simulink model "FRC_0"  (R2018b)
settings: Solver=VariableStepAuto  StartTime=0.0  StopTime=500000.0  RelTol=1e-3
libraries: simulink x1
(part 1 of 2)
settings Model: Creator=user  LastModifiedBy=user

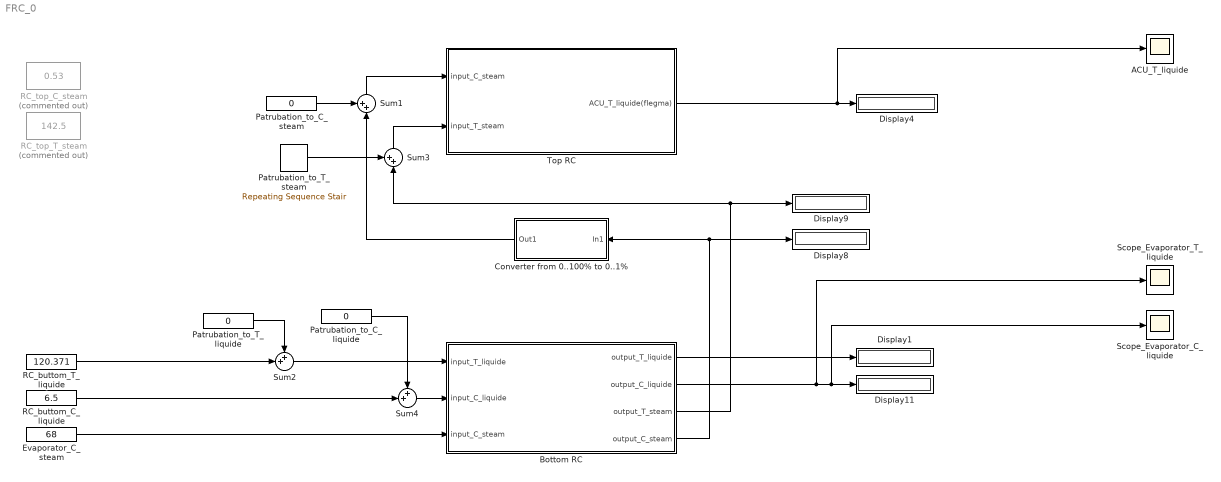
== system FRC_0 ==
  ACU_T_liquide : Scope
  Bottom RC : Subsystem
  Converter from 0..100% to 0..1% : Subsystem
  Display{1,4,8..9,11} (5 alike) : Display
  Evaporator_C_steam : Constant  Value=68
  Patrubation_to_C_liquide : Constant  Value=0
  Patrubation_to_C_steam : Constant  Value=0
  Patrubation_to_T_liquide : Constant  Value=0
  Patrubation_to_T_steam : simulink/Sources/Repeating Sequence Stair  OutValues=[0 0 0 0 0 0 0 0 0 0 2 2 2 2 2 2 2 2].'  tsamp=-1  OutMin=[]  OutMax=[]  OutDataTypeStr=double  OutputDataTypeScalingMode=double  OutDataType=fixdt(0,8)  ConRadixGroup=Best Precision: Vector-wise  OutScaling=2^-12
  RC_buttom_C_liquide : Constant  Value=6.5
  RC_buttom_T_liquide : Constant  Value=120.371
  RC_top_C_steam : Constant  Commented=on  Value=0.53
  RC_top_T_steam : Constant  Commented=on  Value=142.5
  Scope_Evaporator_C_liquide : Scope
  Scope_Evaporator_T_liquide : Scope
  Sum{1..4} (4 alike) : Sum  Inputs=++|
  Top RC : Subsystem
  wires:
  Top RC/1(ACU_T_liquide(flegma)) -> ACU_T_liquide/1, Display4/1
  Bottom RC/2(output_C_liquide) -> Scope_Evaporator_T_liquide/1, Scope_Evaporator_C_liquide/1, Display11/1
  RC_buttom_C_liquide/1 -> Sum4/2
  Evaporator_C_steam/1 -> Bottom RC/3(input_C_steam)
  RC_buttom_T_liquide/1 -> Sum2/2
  Bottom RC/4(output_C_steam) -> Converter from 0..100% to 0..1%/1(In1), Display8/1
  Bottom RC/3(output_T_steam) -> Sum3/2, Display9/1
  Bottom RC/1(output_T_liquide) -> Display1/1
  Converter from 0..100% to 0..1%/1(Out1) -> Sum1/2
  Sum3/1 -> Top RC/2(input_T_steam)
  Patrubation_to_C_steam/1 -> Sum1/1
  Sum1/1 -> Top RC/1(input_C_steam)
  Sum2/1 -> Bottom RC/1(input_T_liquide)
  Patrubation_to_T_liquide/1 -> Sum2/1
  Patrubation_to_C_liquide/1 -> Sum4/1
  Sum4/1 -> Bottom RC/2(input_C_liquide)
  Patrubation_to_T_steam/1 -> Sum3/1

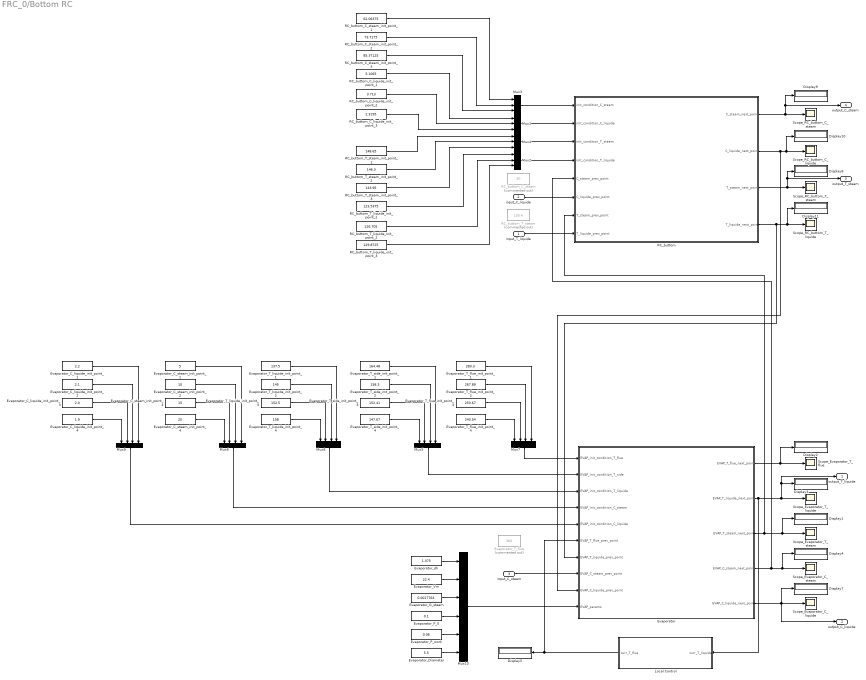
== system FRC_0/Bottom RC ==
  input_T_liquide : Inport
  input_C_liquide : Inport  Port=2
  input_C_steam : Inport  Port=3
  Display{1..5,7..11} (10 alike) : Display
  Evaporator : Subsystem
  Evaporator_C_liquide_init_point_1 : Constant  Value=2.2
  Evaporator_C_liquide_init_point_2 : Constant  Value=2.1
  Evaporator_C_liquide_init_point_3 : Constant  Value=2.0
  Evaporator_C_liquide_init_point_4 : Constant  Value=1.9
  Evaporator_C_steam_init_point_1 : Constant  Value=5
  Evaporator_C_steam_init_point_2 : Constant  Value=10
  Evaporator_C_steam_init_point_3 : Constant  Value=15
  Evaporator_C_steam_init_point_4 : Constant  Value=20
  Evaporator_Diameter : Constant  Value=5.5
  Evaporator_G_steam : Constant  Value=0.0017763
  Evaporator_P_0 : Constant  Value=0.1
  Evaporator_P_work : Constant  Value=0.06
  Evaporator_T_flue : Constant  Commented=on  Value=360
  Evaporator_T_flue_init_point_1 : Constant  Value=283.3
  Evaporator_T_flue_init_point_2 : Constant  Value=267.89
  Evaporator_T_flue_init_point_3 : Constant  Value=253.67
  Evaporator_T_flue_init_point_4 : Constant  Value=240.54
  Evaporator_T_liquide_init_point_1 : Constant  Value=137.5
  Evaporator_T_liquide_init_point_2 : Constant  Value=145
  Evaporator_T_liquide_init_point_3 : Constant  Value=152.5
  Evaporator_T_liquide_init_point_4 : Constant  Value=158
  Evaporator_T_side_init_point_1 : Constant  Value=164.48
  Evaporator_T_side_init_point_2 : Constant  Value=158.3
  Evaporator_T_side_init_point_3 : Constant  Value=152.41
  Evaporator_T_side_init_point_4 : Constant  Value=147.07
  Evaporator_Vm : Constant  Value=22.4
  Evaporator_dh : Constant  Value=1.375
  Local Control : Subsystem
  Mux{1..4} (4 alike) : Mux  Inputs=3
  Mux10 : Mux  Inputs=6
  Mux{5..9} (5 alike) : Mux
  RC_buttom : Subsystem
  RC_buttom_C_liquide_init_point_1 : Constant  Value=5.1065
  RC_buttom_C_liquide_init_point_2 : Constant  Value=3.713
  RC_buttom_C_liquide_init_point_3 : Constant  Value=2.3195
  RC_buttom_C_steam : Constant  Commented=on  Value=50
  RC_buttom_C_steam_init_point_1 : Constant  Value=62.06375
  RC_buttom_C_steam_init_point_2 : Constant  Value=73.7175
  RC_buttom_C_steam_init_point_3 : Constant  Value=85.37125
  RC_buttom_T_liquide_init_point_1 : Constant  Value=123.5375
  RC_buttom_T_liquide_init_point_2 : Constant  Value=126.705
  RC_buttom_T_liquide_init_point_3 : Constant  Value=129.8725
  RC_buttom_T_steam : Constant  Commented=on  Value=150.4
  RC_buttom_T_steam_init_point_1 : Constant  Value=148.65
  RC_buttom_T_steam_init_point_2 : Constant  Value=146.3
  RC_buttom_T_steam_init_point_3 : Constant  Value=143.95
  Scope_Evaporator_C_liquide : Scope
  Scope_Evaporator_C_steam : Scope
  Scope_Evaporator_T_flue : Scope
  Scope_Evaporator_T_liquide : Scope
  Scope_Evaporator_T_steam : Scope
  Scope_RC_buttom_C_liquide : Scope
  Scope_RC_buttom_C_steam : Scope
  Scope_RC_buttom_T_liquide : Scope
  Scope_RC_buttom_T_steam : Scope
  output_T_liquide : Outport
  output_C_liquide : Outport  Port=2
  output_T_steam : Outport  Port=3
  output_C_steam : Outport  Port=4
  wires:
  Evaporator_T_side_init_point_3/1 -> Mux5/2
  Evaporator_C_steam_init_point_2/1 -> Mux6/3
  Evaporator_C_liquide_init_point_1/1 -> Mux9/4
  RC_buttom_T_steam_init_point_1/1 -> Mux4/1
  Evaporator_C_steam_init_point_4/1 -> Mux6/1
  RC_buttom_C_steam_init_point_1/1 -> Mux3/1
  Mux1/1 -> RC_buttom/2(init_condition_C_liquide)
  Evaporator_T_liquide_init_point_4/1 -> Mux8/1
  Evaporator_C_steam_init_point_3/1 -> Mux6/2
  Evaporator/2(EVAP_T_liquide_next_point) -> Local Control/1(curr_T_liquide), output_T_liquide/1, Display3/1, Scope_Evaporator_T_liquide/1
  RC_buttom/4(T_liquide_next_point) -> Evaporator/7(EVAP_T_liquide_prev_point), Display11/1, Scope_RC_buttom_T_liquide/1
  Evaporator_C_liquide_init_point_2/1 -> Mux9/3
  Evaporator_G_steam/1 -> Mux10/3
  Local Control/1(curr_T_flue) -> Evaporator/6(EVAP_T_flue_prev_point), Display5/1
  Mux8/1 -> Evaporator/3(EVAP_init_condition_T_liquide)
  Evaporator_P_0/1 -> Mux10/4
  Mux6/1 -> Evaporator/4(EVAP_init_condition_C_steam)
  Evaporator_T_flue_init_point_2/1 -> Mux7/3
  RC_buttom_C_liquide_init_point_2/1 -> Mux1/2
  Evaporator_P_work/1 -> Mux10/5
  RC_buttom_T_steam_init_point_3/1 -> Mux4/3
  Evaporator_C_liquide_init_point_3/1 -> Mux9/2
  Evaporator_C_liquide_init_point_4/1 -> Mux9/1
  input_T_liquide/1 -> RC_buttom/8(T_liquide_prev_point)
  Mux4/1 -> RC_buttom/3(init_condition_T_steam)
  Evaporator/1(EVAP_T_flue_next_point) -> Display2/1, Scope_Evaporator_T_flue/1
  Evaporator_T_flue_init_point_4/1 -> Mux7/1
  RC_buttom/3(T_steam_next_point) -> output_T_steam/1, Display8/1, Scope_RC_buttom_T_steam/1
  Evaporator/3(EVAP_T_steam_next_point) -> Display1/1, Scope_Evaporator_T_steam/1, RC_buttom/7(T_steam_prev_point)
  RC_buttom_C_liquide_init_point_1/1 -> Mux1/1
  Evaporator_T_flue_init_point_1/1 -> Mux7/4
  RC_buttom/2(C_liquide_next_point) -> Display10/1, Scope_RC_buttom_C_liquide/1, Evaporator/9(EVAP_C_liquide_prev_point)
  Evaporator/5(EVAP_C_liquide_next_point) -> output_C_liquide/1, Display7/1, Scope_Evaporator_C_liquide/1
  Mux3/1 -> RC_buttom/1(init_condition_C_steam)
  Evaporator_T_side_init_point_1/1 -> Mux5/4
  RC_buttom_T_steam_init_point_2/1 -> Mux4/2
  RC_buttom_C_steam_init_point_2/1 -> Mux3/2
  Evaporator_T_side_init_point_2/1 -> Mux5/3
  RC_buttom_T_liquide_init_point_1/1 -> Mux2/1
  Evaporator_T_side_init_point_4/1 -> Mux5/1
  Evaporator_T_flue_init_point_3/1 -> Mux7/2
  RC_buttom_C_liquide_init_point_3/1 -> Mux1/3
  Evaporator_T_liquide_init_point_1/1 -> Mux8/4
  RC_buttom_T_liquide_init_point_3/1 -> Mux2/3
  RC_buttom/1(C_steam_next_point) -> Display9/1, output_C_steam/1, Scope_RC_buttom_C_steam/1
  Evaporator_T_liquide_init_point_2/1 -> Mux8/3
  Evaporator_Vm/1 -> Mux10/2
  Mux7/1 -> Evaporator/1(EVAP_init_condition_T_flue)
  RC_buttom_T_liquide_init_point_2/1 -> Mux2/2
  Mux5/1 -> Evaporator/2(EVAP_init_condition_T_side)
  input_C_steam/1 -> Evaporator/8(EVAP_C_steam_prev_point)
  Mux2/1 -> RC_buttom/4(init_condition_T_liquide)
  Evaporator/4(EVAP_C_steam_next_point) -> RC_buttom/5(C_steam_prev_point), Display4/1, Scope_Evaporator_C_steam/1
  Mux10/1 -> Evaporator/10(EVAP_params)
  Evaporator_C_steam_init_point_1/1 -> Mux6/4
  Evaporator_T_liquide_init_point_3/1 -> Mux8/2
  Mux9/1 -> Evaporator/5(EVAP_init_condition_C_liquide)
  RC_buttom_C_steam_init_point_3/1 -> Mux3/3
  Evaporator_dh/1 -> Mux10/1
  Evaporator_Diameter/1 -> Mux10/6
  input_C_liquide/1 -> RC_buttom/6(C_liquide_prev_point)

== system FRC_0/Converter from 0..100% to 0..1% ==
  In1 : Inport
  Converter from 0..100% to 0..1% : Gain  Gain=0.01
  Out1 : Outport
  wires:
  In1/1 -> Converter from 0..100% to 0..1%/1
  Converter from 0..100% to 0..1%/1 -> Out1/1

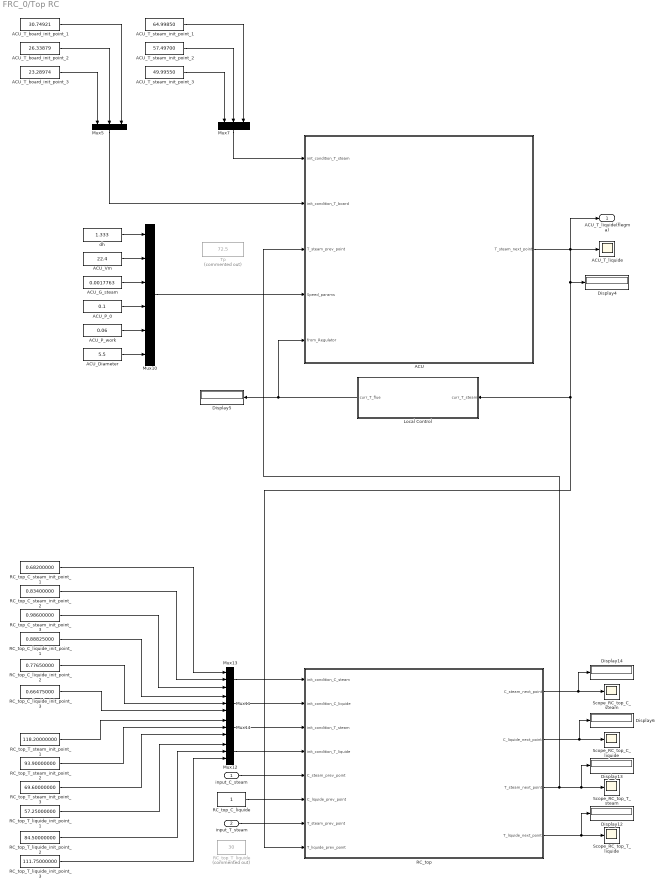
== system FRC_0/Top RC ==
  input_C_steam : Inport
  input_T_steam : Inport  Port=2
  ACU : Subsystem
  ACU_Diameter : Constant  Value=5.5
  ACU_G_steam : Constant  Value=0.0017763
  ACU_P_0 : Constant  Value=0.1
  ACU_P_work : Constant  Value=0.06
  ACU_T_board_init_point_1 : Constant  Value=30.74921
  ACU_T_board_init_point_2 : Constant  Value=26.33879
  ACU_T_board_init_point_3 : Constant  Value=23.28974
  ACU_T_liquide : Scope
  ACU_T_steam_init_point_1 : Constant  Value=64.99850
  ACU_T_steam_init_point_2 : Constant  Value=57.49700
  ACU_T_steam_init_point_3 : Constant  Value=49.99550
  ACU_Vm : Constant  Value=22.4
  Display{4..6,12..14} (6 alike) : Display
  Local Control : Subsystem
  Mux10 : Mux  Inputs=6
  Mux{5,7,11..14} (6 alike) : Mux  Inputs=3
  RC_top : Subsystem
  RC_top_C_liquide : Constant
  RC_top_C_liquide_init_point_1 : Constant  Value=0.88825000
  RC_top_C_liquide_init_point_2 : Constant  Value=0.77650000
  RC_top_C_liquide_init_point_3 : Constant  Value=0.66475000
  RC_top_C_steam_init_point_1 : Constant  Value=0.68200000
  RC_top_C_steam_init_point_2 : Constant  Value=0.83400000
  RC_top_C_steam_init_point_3 : Constant  Value=0.98600000
  RC_top_T_liquide : Constant  Commented=on  Value=30
  RC_top_T_liquide_init_point_1 : Constant  Value=57.25000000
  RC_top_T_liquide_init_point_2 : Constant  Value=84.50000000
  RC_top_T_liquide_init_point_3 : Constant  Value=111.75000000
  RC_top_T_steam_init_point_1 : Constant  Value=118.20000000
  RC_top_T_steam_init_point_2 : Constant  Value=93.90000000
  RC_top_T_steam_init_point_3 : Constant  Value=69.60000000
  Scope_RC_top_C_liquide : Scope
  Scope_RC_top_C_steam : Scope
  Scope_RC_top_T_liquide : Scope
  Scope_RC_top_T_steam : Scope
  Tp : Constant  Commented=on  Value=72.5
  dh : Constant  Value=1.333
  ACU_T_liquide(flegma) : Outport
  wires:
  RC_top_C_steam_init_point_3/1 -> Mux13/3
  RC_top_T_steam_init_point_3/1 -> Mux14/3
  RC_top_T_liquide_init_point_2/1 -> Mux12/2
  RC_top_C_steam_init_point_2/1 -> Mux13/2
  RC_top_C_liquide_init_point_2/1 -> Mux11/2
  RC_top_T_liquide_init_point_1/1 -> Mux12/1
  RC_top/1(C_steam_next_point) -> Display14/1, Scope_RC_top_C_steam/1
  RC_top_C_liquide_init_point_1/1 -> Mux11/1
  Mux14/1 -> RC_top/3(init_condition_T_steam)
  RC_top_C_liquide/1 -> RC_top/6(C_liquide_prev_point)
  RC_top/2(C_liquide_next_point) -> Display6/1, Scope_RC_top_C_liquide/1
  Mux12/1 -> RC_top/4(init_condition_T_liquide)
  RC_top_T_steam_init_point_2/1 -> Mux14/2
  Mux13/1 -> RC_top/1(init_condition_C_steam)
  RC_top_T_liquide_init_point_3/1 -> Mux12/3
  RC_top_T_steam_init_point_1/1 -> Mux14/1
  RC_top_C_liquide_init_point_3/1 -> Mux11/3
  Mux11/1 -> RC_top/2(init_condition_C_liquide)
  RC_top_C_steam_init_point_1/1 -> Mux13/1
  RC_top/4(T_liquide_next_point) -> Display12/1, Scope_RC_top_T_liquide/1
  Mux5/1 -> ACU/2(init_condition_T_board)
  ACU_Vm/1 -> Mux10/2
  Mux7/1 -> ACU/1(init_condition_T_steam)
  ACU_G_steam/1 -> Mux10/3
  ACU_P_work/1 -> Mux10/5
  Local Control/1(curr_T_flue) -> ACU/5(from_Regulator), Display5/1
  ACU_P_0/1 -> Mux10/4
  Mux10/1 -> ACU/4(Speed_params)
  dh/1 -> Mux10/1
  ACU_Diameter/1 -> Mux10/6
  input_C_steam/1 -> RC_top/5(C_steam_prev_point)
  input_T_steam/1 -> RC_top/7(T_steam_prev_point)
  ACU_T_steam_init_point_1/1 -> Mux7/3
  ACU_T_steam_init_point_2/1 -> Mux7/2
  ACU_T_steam_init_point_3/1 -> Mux7/1
  ACU_T_board_init_point_1/1 -> Mux5/3
  ACU_T_board_init_point_2/1 -> Mux5/2
  ACU_T_board_init_point_3/1 -> Mux5/1
  RC_top/3(T_steam_next_point) -> ACU/3(T_steam_prev_point), Display13/1, Scope_RC_top_T_steam/1
  ACU/1(T_steam_next_point) -> ACU_T_liquide(flegma)/1, RC_top/8(T_liquide_prev_point), Local Control/1(curr_T_steam), Display4/1, ACU_T_liquide/1

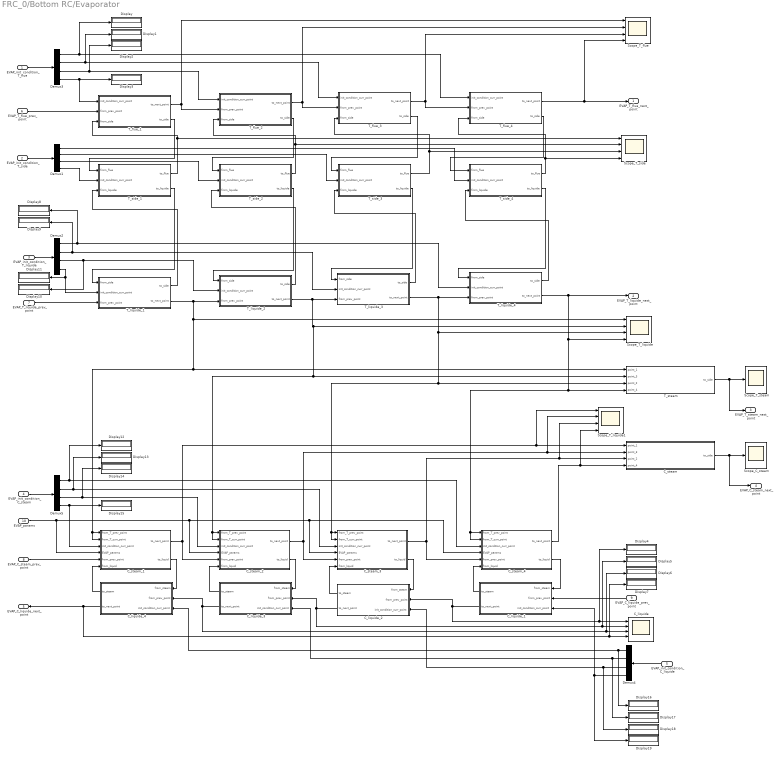
== system FRC_0/Bottom RC/Evaporator ==
  EVAP_init_condition_T_flue : Inport
  EVAP_init_condition_T_side : Inport  Port=2
  EVAP_init_condition_T_liquide : Inport  Port=3
  EVAP_init_condition_C_steam : Inport  Port=4
  EVAP_init_condition_C_liquide : Inport  Port=5
  EVAP_T_flue_prev_point : Inport  Port=6
  EVAP_T_liquide_prev_point : Inport  Port=7
  EVAP_C_steam_prev_point : Inport  Port=8
  EVAP_C_liquide_prev_point : Inport  Port=9
  EVAP_params : Inport  Port=10
  C_liquide : Scope  NumInputPorts=4
  C_liquide_1 : Subsystem
  C_liquide_2 : Subsystem
  C_liquide_3 : Subsystem
  C_liquide_4 : Subsystem
  C_steam : Subsystem
  C_steam_1 : Subsystem
  C_steam_2 : Subsystem
  C_steam_3 : Subsystem
  C_steam_4 : Subsystem
  Demux{1..5} (5 alike) : Demux
  Display{,1..19} (20 alike) : Display
  Scope_C_steam : Scope
  Scope_T_flue : Scope  NumInputPorts=4
  Scope_T_liquide : Scope  NumInputPorts=4
  Scope_T_liquide1 : Scope  NumInputPorts=4
  Scope_T_side : Scope  NumInputPorts=4
  Scope_T_steam : Scope
  T_flue_1 : Subsystem
  T_flue_2 : Subsystem
  T_flue_3 : Subsystem
  T_flue_4 : Subsystem
  T_liquide_1 : Subsystem
  T_liquide_2 : Subsystem
  T_liquide_3 : Subsystem
  T_liquide_4 : Subsystem
  T_side_1 : Subsystem
  T_side_2 : Subsystem
  T_side_3 : Subsystem
  T_side_4 : Subsystem
  T_steam : Subsystem
  EVAP_T_flue_next_point : Outport
  EVAP_T_liquide_next_point : Outport  Port=2
  EVAP_T_steam_next_point : Outport  Port=3
  EVAP_C_steam_next_point : Outport  Port=4
  EVAP_C_liquide_next_point : Outport  Port=5
  wires:
  T_liquide_3/2(to_next_point) -> T_liquide_4/3(from_prev_point), C_steam_3/1(from_T_prev_point), C_steam_3/2(from_T_curr_point), T_steam/3(point_2), Scope_T_liquide/3
  EVAP_init_condition_T_liquide/1 -> Demux2/1
  Demux2/1 -> T_liquide_4/2(init_condition_curr_point), Display8/1
  EVAP_init_condition_T_side/1 -> Demux1/1
  T_liquide_4/2(to_next_point) -> Scope_T_liquide/4, C_steam_4/2(from_T_curr_point), C_steam_4/1(from_T_prev_point), T_steam/4(point_4), EVAP_T_liquide_next_point/1
  Demux2/2 -> T_liquide_3/2(init_condition_curr_point), Display9/1
  Demux2/4 -> T_liquide_1/2(init_condition_curr_point), Display11/1
  EVAP_init_condition_T_flue/1 -> Demux3/1
  T_flue_1/1(to_next_point) -> T_flue_2/2(from_prev_point), Scope_T_flue/1
  T_flue_2/1(to_next_point) -> T_flue_3/2(from_prev_point), Scope_T_flue/2
  T_flue_3/1(to_next_point) -> T_flue_4/2(from_prev_point), Scope_T_flue/3
  Demux3/1 -> T_flue_4/1(init_condition_curr_point), Display/1
  Demux3/2 -> T_flue_3/1(init_condition_curr_point), Display1/1
  Demux3/3 -> T_flue_2/1(init_condition_curr_point), Display2/1
  Demux3/4 -> T_flue_1/1(init_condition_curr_point), Display3/1
  T_flue_4/1(to_next_point) -> EVAP_T_flue_next_point/1, Scope_T_flue/4
  EVAP_T_flue_prev_point/1 -> T_flue_1/2(from_prev_point)
  T_steam/1(to_side) -> EVAP_T_steam_next_point/1, Scope_T_steam/1
  Demux5/2 -> C_steam_3/3(init_condition_curr_point), Display13/1
  C_liquide_2/2(to_next_point) -> C_liquide_3/2(from_prev_point), Display5/1, C_liquide/2
  C_steam_2/1(to_next_point) -> C_steam_3/5(from_prev_point), Scope_T_liquide1/2, C_steam/2(point_3)
  EVAP_init_condition_C_liquide/1 -> Demux4/1
  Demux5/3 -> C_steam_2/3(init_condition_curr_point), Display14/1
  C_steam_1/2(to_liquid) -> C_liquide_4/1(from_steam)
  Demux5/1 -> C_steam_4/3(init_condition_curr_point), Display12/1
  EVAP_init_condition_C_steam/1 -> Demux5/1
  EVAP_C_steam_prev_point/1 -> C_steam_1/5(from_prev_point)
  C_liquide_4/2(to_next_point) -> EVAP_C_liquide_next_point/1, Display7/1, C_liquide/4
  C_liquide_2/1(to_steam) -> C_steam_3/6(from_liquid)
  C_liquide_3/2(to_next_point) -> C_liquide_4/2(from_prev_point), Display6/1, C_liquide/3
  C_liquide_4/1(to_steam) -> C_steam_1/6(from_liquid)
  C_steam_3/1(to_next_point) -> C_steam_4/5(from_prev_point), Scope_T_liquide1/3, C_steam/3(point_2)
  EVAP_C_liquide_prev_point/1 -> C_liquide_1/2(from_prev_point)
  C_steam_4/2(to_liquid) -> C_liquide_1/1(from_steam)
  C_liquide_1/1(to_steam) -> C_steam_4/6(from_liquid)
  Demux5/4 -> C_steam_1/3(init_condition_curr_point), Display15/1
  C_liquide_1/2(to_next_point) -> C_liquide_2/2(from_prev_point), Display4/1, C_liquide/1
  Demux4/1 -> C_liquide_4/3(init_condition_curr_point), Display16/1
  Demux4/2 -> C_liquide_3/3(init_condition_curr_point), Display17/1
  Demux4/3 -> C_liquide_2/3(init_condition_curr_point), Display18/1
  Demux4/4 -> C_liquide_1/3(init_condition_curr_point), Display19/1
  C_steam/1(to_side) -> EVAP_C_steam_next_point/1, Scope_C_steam/1
  C_steam_1/1(to_next_point) -> C_steam_2/5(from_prev_point), Scope_T_liquide1/1, C_steam/1(point_1)
  C_steam_4/1(to_next_point) -> Scope_T_liquide1/4, C_steam/4(point_4)
  EVAP_params/1 -> C_steam_1/4(EVAP_params), C_steam_2/4(EVAP_params), C_steam_4/4(EVAP_params), C_steam_3/4(EVAP_params)
  C_liquide_3/1(to_steam) -> C_steam_2/6(from_liquid)
  C_steam_2/2(to_liquid) -> C_liquide_3/1(from_steam)
  EVAP_T_liquide_prev_point/1 -> T_liquide_1/3(from_prev_point)
  C_steam_3/2(to_liquid) -> C_liquide_2/1(from_steam)
  T_liquide_1/2(to_next_point) -> T_liquide_2/3(from_prev_point), Scope_T_liquide/1, T_steam/1(point_1), C_steam_1/1(from_T_prev_point), C_steam_1/2(from_T_curr_point)
  Demux2/3 -> T_liquide_2/2(init_condition_curr_point), Display10/1
  T_side_1/1(to_flue) -> Scope_T_side/1, T_flue_1/3(from_side)
  T_flue_1/2(to_side) -> T_side_1/1(from_flue)
  T_side_1/2(to_liquide) -> T_liquide_1/1(from_side)
  T_liquide_1/1(to_side) -> T_side_1/3(from_liquide)
  Demux1/4 -> T_side_1/2(init_condition_curr_point)
  T_side_2/1(to_flue) -> T_flue_2/3(from_side), Scope_T_side/2
  T_flue_2/2(to_side) -> T_side_2/1(from_flue)
  T_side_3/1(to_flue) -> T_flue_3/3(from_side), Scope_T_side/3
  T_flue_3/2(to_side) -> T_side_3/1(from_flue)
  T_side_4/1(to_flue) -> T_flue_4/3(from_side), Scope_T_side/4
  T_flue_4/2(to_side) -> T_side_4/1(from_flue)
  T_liquide_2/1(to_side) -> T_side_2/3(from_liquide)
  T_side_2/2(to_liquide) -> T_liquide_2/1(from_side)
  T_side_3/2(to_liquide) -> T_liquide_3/1(from_side)
  T_liquide_3/1(to_side) -> T_side_3/3(from_liquide)
  T_side_4/2(to_liquide) -> T_liquide_4/1(from_side)
  T_liquide_4/1(to_side) -> T_side_4/3(from_liquide)
  Demux1/3 -> T_side_2/2(init_condition_curr_point)
  Demux1/2 -> T_side_3/2(init_condition_curr_point)
  Demux1/1 -> T_side_4/2(init_condition_curr_point)
  T_liquide_2/2(to_next_point) -> T_liquide_3/3(from_prev_point), C_steam_2/2(from_T_curr_point), C_steam_2/1(from_T_prev_point), T_steam/2(point_3), Scope_T_liquide/2

== system FRC_0/Bottom RC/Local Control ==
  curr_T_liquide : Inport
  %/c : RateLimiter  RisingSlewLimit=5  FallingSlewLimit=-5  SampleTimeMode=inherited
  Display2 : Display
  "Kdta, mA/C" : Gain  Gain=0.08
  Kpi : Gain
  Kro : Gain  Gain=0.006
  "Kzd, mA/C" : Gain  Gain=0.08
  Sum29 : Sum  Inputs=+-
  Sum30 : Sum
  Ti : Integrator  InitialCondition=8000  UpperSaturationLimit=8012  LowerSaturationLimit=6012
  "Tz, C" : Constant  Value=160.00
  "pozicioner, %/mA" : Gain  Gain=6.25
  curr_T_flue : Outport
  wires:
  Ti/1 -> Sum30/2
  Kpi/1 -> Ti/1, Sum30/1
  "Tz, C"/1 -> "Kzd, mA/C"/1
  "Kzd, mA/C"/1 -> Sum29/1
  %/c/1 -> Kro/1
  "Kdta, mA/C"/1 -> Sum29/2
  curr_T_liquide/1 -> "Kdta, mA/C"/1
  "pozicioner, %/mA"/1 -> %/c/1
  Sum30/1 -> "pozicioner, %/mA"/1
  Kro/1 -> curr_T_flue/1, Display2/1
  Sum29/1 -> Kpi/1

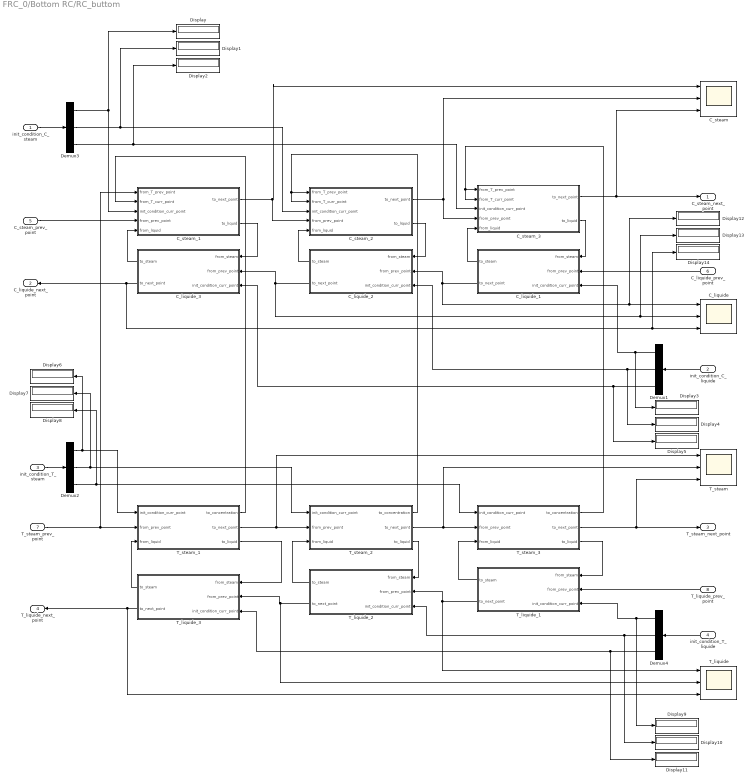
== system FRC_0/Bottom RC/RC_buttom ==
  init_condition_C_steam : Inport
  init_condition_C_liquide : Inport  Port=2
  init_condition_T_steam : Inport  Port=3
  init_condition_T_liquide : Inport  Port=4
  C_steam_prev_point : Inport  Port=5
  C_liquide_prev_point : Inport  Port=6
  T_steam_prev_point : Inport  Port=7
  T_liquide_prev_point : Inport  Port=8
  C_liquide : Scope  NumInputPorts=3
  C_liquide_1 : Subsystem
  C_liquide_2 : Subsystem
  C_liquide_3 : Subsystem
  C_steam : Scope  NumInputPorts=3
  C_steam_1 : Subsystem
  C_steam_2 : Subsystem
  C_steam_3 : Subsystem
  Demux{1..4} (4 alike) : Demux  Outputs=3
  Display{,1..14} (15 alike) : Display
  T_liquide : Scope  NumInputPorts=3
  T_liquide_1 : Subsystem
  T_liquide_2 : Subsystem
  T_liquide_3 : Subsystem
  T_steam : Scope  NumInputPorts=3
  T_steam_1 : Subsystem
  T_steam_2 : Subsystem
  T_steam_3 : Subsystem
  C_steam_next_point : Outport
  C_liquide_next_point : Outport  Port=2
  T_steam_next_point : Outport  Port=3
  T_liquide_next_point : Outport  Port=4
  wires:
  T_steam_2/2(to_next_point) -> T_steam/2, T_steam_3/2(from_prev_point)
  T_steam_3/2(to_next_point) -> T_steam_next_point/1, T_steam/3
  T_steam_prev_point/1 -> C_steam_1/1(from_T_prev_point), T_steam_1/2(from_prev_point)
  T_liquide_1/1(to_steam) -> T_steam_3/3(from_liquid)
  T_steam_3/3(to_liquid) -> T_liquide_1/1(from_steam)
  T_liquide_prev_point/1 -> T_liquide_1/2(from_prev_point)
  T_liquide_1/2(to_next_point) -> T_liquide_2/2(from_prev_point), T_liquide/1
  T_steam_2/3(to_liquid) -> T_liquide_2/1(from_steam)
  T_liquide_2/1(to_steam) -> T_steam_2/3(from_liquid)
  T_liquide_2/2(to_next_point) -> T_liquide_3/2(from_prev_point), T_liquide/2
  T_steam_1/3(to_liquid) -> T_liquide_3/1(from_steam)
  T_liquide_3/1(to_steam) -> T_steam_1/3(from_liquid)
  Demux4/2 -> Display10/1, T_liquide_2/3(init_condition_curr_point)
  Demux4/3 -> Display11/1, T_liquide_3/3(init_condition_curr_point)
  T_liquide_3/2(to_next_point) -> T_liquide/3, T_liquide_next_point/1
  C_liquide_3/1(to_steam) -> C_steam_1/5(from_liquid)
  C_steam_3/1(to_next_point) -> C_steam/3, C_steam_next_point/1
  C_steam_1/1(to_next_point) -> C_steam_2/4(from_prev_point), C_steam/1
  Demux3/3 -> C_steam_3/3(init_condition_curr_point), Display2/1
  C_steam_3/2(to_liquid) -> C_liquide_1/1(from_steam)
  C_liquide_prev_point/1 -> C_liquide_1/2(from_prev_point)
  C_liquide_2/2(to_next_point) -> C_liquide_3/2(from_prev_point), Display13/1, C_liquide/2
  C_steam_2/2(to_liquid) -> C_liquide_2/1(from_steam)
  C_liquide_1/1(to_steam) -> C_steam_3/5(from_liquid)
  C_liquide_3/2(to_next_point) -> Display14/1, C_liquide/3, C_liquide_next_point/1
  Demux1/2 -> C_liquide_2/3(init_condition_curr_point), Display4/1
  Demux1/3 -> C_liquide_3/3(init_condition_curr_point), Display5/1
  C_steam_prev_point/1 -> C_steam_1/4(from_prev_point)
  C_steam_1/2(to_liquid) -> C_liquide_3/1(from_steam)
  C_liquide_2/1(to_steam) -> C_steam_2/5(from_liquid)
  C_liquide_1/2(to_next_point) -> C_liquide_2/2(from_prev_point), Display12/1, C_liquide/1
  init_condition_T_steam/1 -> Demux2/1
  Demux2/1 -> T_steam_1/1(init_condition_curr_point), Display6/1
  Demux2/3 -> T_steam_3/1(init_condition_curr_point), Display8/1
  init_condition_T_liquide/1 -> Demux4/1
  Demux4/1 -> Display9/1, T_liquide_1/3(init_condition_curr_point)
  init_condition_C_steam/1 -> Demux3/1
  Demux3/2 -> C_steam_2/3(init_condition_curr_point), Display1/1
  init_condition_C_liquide/1 -> Demux1/1
  Demux1/1 -> C_liquide_1/3(init_condition_curr_point), Display3/1
  C_steam_2/1(to_next_point) -> C_steam/2, C_steam_3/4(from_prev_point)
  T_steam_2/1(to_concentration) -> C_steam_2/1(from_T_prev_point), C_steam_2/2(from_T_curr_point)
  T_steam_3/1(to_concentration) -> C_steam_3/1(from_T_prev_point), C_steam_3/2(from_T_curr_point)
  Demux2/2 -> T_steam_2/1(init_condition_curr_point), Display7/1
  T_steam_1/2(to_next_point) -> T_steam/1, T_steam_2/2(from_prev_point)
  Demux3/1 -> Display/1, C_steam_1/3(init_condition_curr_point)
  T_steam_1/1(to_concentration) -> C_steam_1/2(from_T_curr_point)

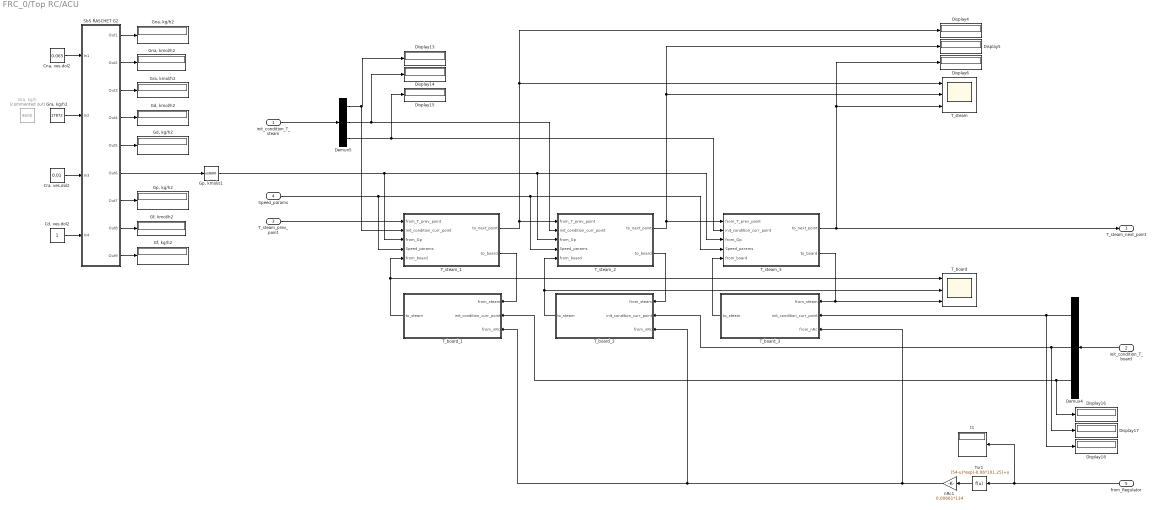
== system FRC_0/Top RC/ACU ==
  init_condition_T_steam : Inport
  init_condition_T_board : Inport  Port=2
  T_steam_prev_point : Inport  Port=3
  Speed_params : Inport  Port=4
  from_Regulator : Inport  Port=5
  "Cd, ves.dol2" : Constant
  "Cna, ves.dol2" : Constant  Value=0.065
  "Cra, ves.dol2" : Constant  Value=0.01
  Demux4 : Demux  Outputs=3
  Demux5 : Demux  Outputs=3
  Display{4..6,13..18} (9 alike) : Display
  "Gd, kg/h2" : Display
  "Gd, kmol/h2" : Display
  "Gf, kg/h2" : Display
  "Gf, kmol/h2" : Display
  "Gna, kg/h2" : Display
  "Gna, kmol/h2" : Display
  "Gp, kmol/s1" : Fcn  Expr=u/3600
  "Gp, kg/h2" : Display
  "Gra, kg/h" : Constant  Commented=on  Value=9600
  "Gra, kg/h2" : Constant  Value=17872
  "Gra, kmol/h2" : Display
  SbS RASCHET G2 : Subsystem
  T_board : Scope  NumInputPorts=3
  T_board_1 : Subsystem
  T_board_2 : Subsystem
  T_board_3 : Subsystem
  T_steam : Scope  NumInputPorts=3
  T_steam_1 : Subsystem
  T_steam_2 : Subsystem
  T_steam_3 : Subsystem
  Tsr1 : Fcn  Expr=(54-u)*exp(-0.06*101.25)+u
  nRc1 : Gain  Gain=0.00661*134
  t1 : Display
  T_steam_next_point : Outport
  wires:
  T_steam_2/1(to_next_point) -> T_steam_3/1(from_T_prev_point), Display5/1, T_steam/2
  init_condition_T_board/1 -> Demux4/1
  init_condition_T_steam/1 -> Demux5/1
  T_steam_3/1(to_next_point) -> T_steam_next_point/1, Display6/1, T_steam/3
  T_steam_1/1(to_next_point) -> T_steam/1, Display4/1, T_steam_2/1(from_T_prev_point)
  Speed_params/1 -> T_steam_2/4(Speed_params), T_steam_3/4(Speed_params), T_steam_1/4(Speed_params)
  "Cd, ves.dol2"/1 -> SbS RASCHET G2/4(In4)
  SbS RASCHET G2/3(Out3) -> "Gra, kmol/h2"/1
  SbS RASCHET G2/9(Out9) -> "Gf, kg/h2"/1
  SbS RASCHET G2/1(Out1) -> "Gna, kg/h2"/1
  SbS RASCHET G2/5(Out5) -> "Gd, kg/h2"/1
  SbS RASCHET G2/7(Out7) -> "Gp, kg/h2"/1
  SbS RASCHET G2/2(Out2) -> "Gna, kmol/h2"/1
  "Gra, kg/h2"/1 -> SbS RASCHET G2/2(In2)
  SbS RASCHET G2/4(Out4) -> "Gd, kmol/h2"/1
  "Cra, ves.dol2"/1 -> SbS RASCHET G2/3(In3)
  "Cna, ves.dol2"/1 -> SbS RASCHET G2/1(In1)
  SbS RASCHET G2/8(Out8) -> "Gf, kmol/h2"/1
  SbS RASCHET G2/6(Out6) -> "Gp, kmol/s1"/1
  T_steam_prev_point/1 -> T_steam_1/1(from_T_prev_point)
  "Gp, kmol/s1"/1 -> T_steam_3/3(from_Gp), T_steam_2/3(from_Gp), T_steam_1/3(from_Gp)
  Tsr1/1 -> nRc1/1
  T_board_1/1(to_steam) -> T_steam_1/5(from_board), T_board/1
  T_steam_1/2(to_board) -> T_board_1/1(from_steam)
  T_board_2/1(to_steam) -> T_steam_2/5(from_board), T_board/2
  T_steam_2/2(to_board) -> T_board_2/1(from_steam)
  T_board_3/1(to_steam) -> T_steam_3/5(from_board)
  T_steam_3/2(to_board) -> T_board/3, T_board_3/1(from_steam)
  nRc1/1 -> T_board_3/3(from_nRc), T_board_2/3(from_nRc), T_board_1/3(from_nRc)
  Demux4/1 -> Display18/1, T_board_3/2(init_condition_curr_point)
  Demux4/2 -> Display17/1, T_board_2/2(init_condition_curr_point)
  Demux4/3 -> Display16/1, T_board_1/2(init_condition_curr_point)
  Demux5/1 -> T_steam_1/2(init_condition_curr_point), Display13/1
  from_Regulator/1 -> t1/1, Tsr1/1
  Demux5/2 -> T_steam_2/2(init_condition_curr_point), Display14/1
  Demux5/3 -> Display15/1, T_steam_3/2(init_condition_curr_point)

== system FRC_0/Top RC/Local Control ==
  curr_T_steam : Inport
  Pr.f : Subsystem
  Sum9 : Sum  Inputs=-+
  Tnpz : Constant  Value=30
  kDT : Gain  Gain=7.717*10^(-5)
  t : Display
  t1 : Display
  curr_T_flue : Outport
  wires:
  kDT/1 -> Pr.f/1(In1)
  Sum9/1 -> kDT/1
  curr_T_steam/1 -> Sum9/1, t/1
  Tnpz/1 -> Sum9/2
  Pr.f/1(Out1) -> curr_T_flue/1, t1/1

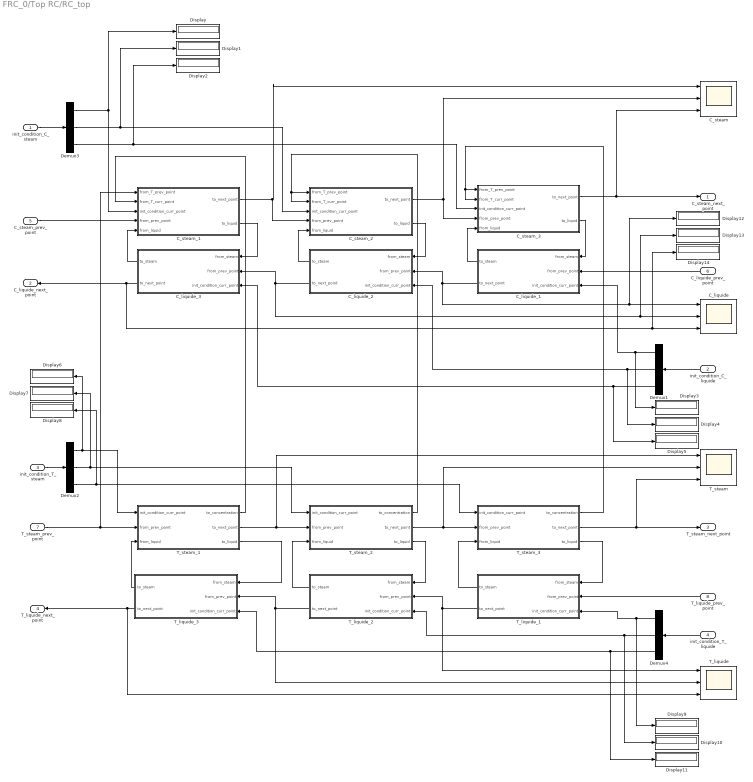
== system FRC_0/Top RC/RC_top ==
  init_condition_C_steam : Inport
  init_condition_C_liquide : Inport  Port=2
  init_condition_T_steam : Inport  Port=3
  init_condition_T_liquide : Inport  Port=4
  C_steam_prev_point : Inport  Port=5
  C_liquide_prev_point : Inport  Port=6
  T_steam_prev_point : Inport  Port=7
  T_liquide_prev_point : Inport  Port=8
  C_liquide : Scope  NumInputPorts=3
  C_liquide_1 : Subsystem
  C_liquide_2 : Subsystem
  C_liquide_3 : Subsystem
  C_steam : Scope  NumInputPorts=3
  C_steam_1 : Subsystem
  C_steam_2 : Subsystem
  C_steam_3 : Subsystem
  Demux{1..4} (4 alike) : Demux  Outputs=3
  Display{,1..14} (15 alike) : Display
  T_liquide : Scope  NumInputPorts=3
  T_liquide_1 : Subsystem
  T_liquide_2 : Subsystem
  T_liquide_3 : Subsystem
  T_steam : Scope  NumInputPorts=3
  T_steam_1 : Subsystem
  T_steam_2 : Subsystem
  T_steam_3 : Subsystem
  C_steam_next_point : Outport
  C_liquide_next_point : Outport  Port=2
  T_steam_next_point : Outport  Port=3
  T_liquide_next_point : Outport  Port=4
  wires:
  T_steam_2/2(to_next_point) -> T_steam_3/2(from_prev_point), T_steam/2
  T_steam_3/2(to_next_point) -> T_steam_next_point/1, T_steam/3
  T_steam_prev_point/1 -> C_steam_1/1(from_T_prev_point), T_steam_1/2(from_prev_point)
  T_liquide_1/1(to_steam) -> T_steam_3/3(from_liquid)
  T_steam_3/3(to_liquid) -> T_liquide_1/1(from_steam)
  T_liquide_prev_point/1 -> T_liquide_1/2(from_prev_point)
  T_liquide_1/2(to_next_point) -> T_liquide_2/2(from_prev_point), T_liquide/1
  T_steam_2/3(to_liquid) -> T_liquide_2/1(from_steam)
  T_liquide_2/1(to_steam) -> T_steam_2/3(from_liquid)
  T_liquide_2/2(to_next_point) -> T_liquide_3/2(from_prev_point), T_liquide/2
  T_steam_1/3(to_liquid) -> T_liquide_3/1(from_steam)
  T_liquide_3/1(to_steam) -> T_steam_1/3(from_liquid)
  Demux4/2 -> T_liquide_2/3(init_condition_curr_point), Display10/1
  Demux4/3 -> T_liquide_3/3(init_condition_curr_point), Display11/1
  T_liquide_3/2(to_next_point) -> T_liquide/3, T_liquide_next_point/1
  C_liquide_3/1(to_steam) -> C_steam_1/5(from_liquid)
  C_steam_3/1(to_next_point) -> C_steam/3, C_steam_next_point/1
  C_steam_1/1(to_next_point) -> C_steam_2/4(from_prev_point), C_steam/1
  Demux3/3 -> C_steam_3/3(init_condition_curr_point), Display2/1
  C_steam_3/2(to_liquid) -> C_liquide_1/1(from_steam)
  C_liquide_prev_point/1 -> C_liquide_1/2(from_prev_point)
  C_liquide_2/2(to_next_point) -> C_liquide_3/2(from_prev_point), Display13/1, C_liquide/2
  C_steam_2/2(to_liquid) -> C_liquide_2/1(from_steam)
  C_liquide_1/1(to_steam) -> C_steam_3/5(from_liquid)
  C_liquide_3/2(to_next_point) -> Display14/1, C_liquide/3, C_liquide_next_point/1
  Demux1/2 -> C_liquide_2/3(init_condition_curr_point), Display4/1
  Demux1/3 -> C_liquide_3/3(init_condition_curr_point), Display5/1
  C_steam_prev_point/1 -> C_steam_1/4(from_prev_point)
  C_steam_1/2(to_liquid) -> C_liquide_3/1(from_steam)
  C_liquide_2/1(to_steam) -> C_steam_2/5(from_liquid)
  C_liquide_1/2(to_next_point) -> C_liquide_2/2(from_prev_point), Display12/1, C_liquide/1
  init_condition_T_steam/1 -> Demux2/1
  Demux2/1 -> T_steam_1/1(init_condition_curr_point), Display6/1
  Demux2/3 -> T_steam_3/1(init_condition_curr_point), Display8/1
  init_condition_T_liquide/1 -> Demux4/1
  Demux4/1 -> Display9/1, T_liquide_1/3(init_condition_curr_point)
  init_condition_C_steam/1 -> Demux3/1
  Demux3/2 -> C_steam_2/3(init_condition_curr_point), Display1/1
  init_condition_C_liquide/1 -> Demux1/1
  Demux1/1 -> C_liquide_1/3(init_condition_curr_point), Display3/1
  C_steam_2/1(to_next_point) -> C_steam_3/4(from_prev_point), C_steam/2
  T_steam_2/1(to_concentration) -> C_steam_2/2(from_T_curr_point), C_steam_2/1(from_T_prev_point)
  T_steam_3/1(to_concentration) -> C_steam_3/2(from_T_curr_point), C_steam_3/1(from_T_prev_point)
  Demux2/2 -> T_steam_2/1(init_condition_curr_point), Display7/1
  T_steam_1/2(to_next_point) -> T_steam_2/2(from_prev_point), T_steam/1
  Demux3/1 -> Display/1, C_steam_1/3(init_condition_curr_point)
  T_steam_1/1(to_concentration) -> C_steam_1/2(from_T_curr_point)

== system FRC_0/Bottom RC/Evaporator/C_liquide_1 ==
  from_steam : Inport
  from_prev_point : Inport  Port=2
  init_condition_curr_point : Inport  Port=3
  Gain18 : Gain  Gain=0.000004000
  Gain19 : Gain  Gain=0.003/1.375
  Gain22 : Gain  Gain=0.003/1.375-(0.000004000)*10^(-9)
  Sum2 : Sum  Inputs=-+-
  Tl1 : Integrator  InitialConditionSource=external  InitialCondition=124.3766
  to_steam : Outport
  to_next_point : Outport  Port=2
  wires:
  from_steam/1 -> Gain18/1
  from_prev_point/1 -> Gain19/1
  Gain19/1 -> Sum2/2
  Sum2/1 -> Tl1/1
  Gain18/1 -> Sum2/1
  init_condition_curr_point/1 -> Tl1/2
  Gain22/1 -> Sum2/3
  Tl1/1 -> Gain22/1, to_steam/1, to_next_point/1

== system FRC_0/Bottom RC/Evaporator/C_liquide_2 ==
  from_steam : Inport
  from_prev_point : Inport  Port=2
  init_condition_curr_point : Inport  Port=3
  Gain18 : Gain  Gain=0.000004000
  Gain19 : Gain  Gain=0.003/1.375
  Gain22 : Gain  Gain=0.003/1.375-(0.000004000)*10^(-9)
  Sum2 : Sum  Inputs=-+-
  Tl1 : Integrator  InitialConditionSource=external  InitialCondition=124.3766
  to_steam : Outport
  to_next_point : Outport  Port=2
  wires:
  from_steam/1 -> Gain18/1
  from_prev_point/1 -> Gain19/1
  Gain19/1 -> Sum2/2
  Sum2/1 -> Tl1/1
  Gain18/1 -> Sum2/1
  init_condition_curr_point/1 -> Tl1/2
  Gain22/1 -> Sum2/3
  Tl1/1 -> Gain22/1, to_steam/1, to_next_point/1

== system FRC_0/Bottom RC/Evaporator/C_liquide_3 ==
  from_steam : Inport
  from_prev_point : Inport  Port=2
  init_condition_curr_point : Inport  Port=3
  Gain18 : Gain  Gain=0.000004000
  Gain19 : Gain  Gain=0.003/1.375
  Gain22 : Gain  Gain=0.003/1.375-(0.000004000)*10^(-9)
  Sum2 : Sum  Inputs=-+-
  Tl1 : Integrator  InitialConditionSource=external  InitialCondition=124.3766
  to_steam : Outport
  to_next_point : Outport  Port=2
  wires:
  from_steam/1 -> Gain18/1
  from_prev_point/1 -> Gain19/1
  Gain19/1 -> Sum2/2
  Sum2/1 -> Tl1/1
  Gain18/1 -> Sum2/1
  init_condition_curr_point/1 -> Tl1/2
  Gain22/1 -> Sum2/3
  Tl1/1 -> Gain22/1, to_steam/1, to_next_point/1

== system FRC_0/Bottom RC/Evaporator/C_liquide_4 ==
  from_steam : Inport
  from_prev_point : Inport  Port=2
  init_condition_curr_point : Inport  Port=3
  Gain18 : Gain  Gain=0.000004000
  Gain19 : Gain  Gain=0.003/1.375
  Gain22 : Gain  Gain=0.003/1.375-(0.000004000)*10^(-9)
  Sum2 : Sum  Inputs=-+-
  Tl1 : Integrator  InitialConditionSource=external  InitialCondition=124.3766
  to_steam : Outport
  to_next_point : Outport  Port=2
  wires:
  from_steam/1 -> Gain18/1
  from_prev_point/1 -> Gain19/1
  Gain19/1 -> Sum2/2
  Sum2/1 -> Tl1/1
  Gain18/1 -> Sum2/1
  init_condition_curr_point/1 -> Tl1/2
  Gain22/1 -> Sum2/3
  Tl1/1 -> Gain22/1, to_steam/1, to_next_point/1

== system FRC_0/Bottom RC/Evaporator/C_steam ==
  point_1 : Inport
  point_3 : Inport  Port=2
  point_2 : Inport  Port=3
  point_4 : Inport  Port=4
  Gain : Gain  Gain=1/4
  Sum37 : Sum  Inputs=++++
  to_side : Outport
  wires:
  point_2/1 -> Sum37/2
  point_1/1 -> Sum37/1
  point_3/1 -> Sum37/3
  point_4/1 -> Sum37/4
  Sum37/1 -> Gain/1
  Gain/1 -> to_side/1

== system FRC_0/Bottom RC/Evaporator/C_steam_1 ==
  from_T_prev_point : Inport
  from_T_curr_point : Inport  Port=2
  init_condition_curr_point : Inport  Port=3
  EVAP_params : Inport  Port=4
  from_prev_point : Inport  Port=5
  from_liquid : Inport  Port=6
  C_steam : Integrator  InitialConditionSource=external  InitialCondition=156.9966
  Gain29 : Gain  Gain=0.0000216487318*10^(-9)
  Sum3 : Sum  Inputs=-+-
  k1 : Subsystem
  speed : Subsystem
  to_next_point : Outport
  to_liquid : Outport  Port=2
  wires:
  init_condition_curr_point/1 -> C_steam/2
  speed/1(Out1) -> Sum3/2
  Gain29/1 -> Sum3/3
  Sum3/1 -> C_steam/1
  from_liquid/1 -> Gain29/1
  k1/1(Out1) -> Sum3/1
  C_steam/1 -> k1/2(In2), to_next_point/1, to_liquid/1
  from_T_curr_point/1 -> k1/1(In1)
  EVAP_params/1 -> k1/3(EVAP_params1), speed/3(EVAP_params)
  from_prev_point/1 -> speed/1(In1)
  from_T_prev_point/1 -> speed/2(In2)

== system FRC_0/Bottom RC/Evaporator/C_steam_2 ==
  from_T_prev_point : Inport
  from_T_curr_point : Inport  Port=2
  init_condition_curr_point : Inport  Port=3
  EVAP_params : Inport  Port=4
  from_prev_point : Inport  Port=5
  from_liquid : Inport  Port=6
  C_steam : Integrator  InitialConditionSource=external  InitialCondition=156.9966
  Gain29 : Gain  Gain=0.0000216487318*10^(-9)
  Sum3 : Sum  Inputs=-+-
  k1 : Subsystem
  speed : Subsystem
  to_next_point : Outport
  to_liquid : Outport  Port=2
  wires:
  init_condition_curr_point/1 -> C_steam/2
  speed/1(Out1) -> Sum3/2
  Gain29/1 -> Sum3/3
  Sum3/1 -> C_steam/1
  from_liquid/1 -> Gain29/1
  k1/1(Out1) -> Sum3/1
  C_steam/1 -> k1/2(In2), to_next_point/1, to_liquid/1
  from_T_curr_point/1 -> k1/1(In1)
  EVAP_params/1 -> k1/3(EVAP_params1), speed/3(EVAP_params)
  from_prev_point/1 -> speed/1(In1)
  from_T_prev_point/1 -> speed/2(In2)

== system FRC_0/Bottom RC/Evaporator/C_steam_3 ==
  from_T_prev_point : Inport
  from_T_curr_point : Inport  Port=2
  init_condition_curr_point : Inport  Port=3
  EVAP_params : Inport  Port=4
  from_prev_point : Inport  Port=5
  from_liquid : Inport  Port=6
  C_steam : Integrator  InitialConditionSource=external  InitialCondition=156.9966
  Gain29 : Gain  Gain=0.0000216487318*10^(-9)
  Sum3 : Sum  Inputs=-+-
  k1 : Subsystem
  speed : Subsystem
  to_next_point : Outport
  to_liquid : Outport  Port=2
  wires:
  init_condition_curr_point/1 -> C_steam/2
  speed/1(Out1) -> Sum3/2
  Gain29/1 -> Sum3/3
  Sum3/1 -> C_steam/1
  from_liquid/1 -> Gain29/1
  k1/1(Out1) -> Sum3/1
  C_steam/1 -> k1/2(In2), to_next_point/1, to_liquid/1
  from_T_curr_point/1 -> k1/1(In1)
  EVAP_params/1 -> k1/3(EVAP_params1), speed/3(EVAP_params)
  from_prev_point/1 -> speed/1(In1)
  from_T_prev_point/1 -> speed/2(In2)

== system FRC_0/Bottom RC/Evaporator/C_steam_4 ==
  from_T_prev_point : Inport
  from_T_curr_point : Inport  Port=2
  init_condition_curr_point : Inport  Port=3
  EVAP_params : Inport  Port=4
  from_prev_point : Inport  Port=5
  from_liquid : Inport  Port=6
  C_steam : Integrator  InitialConditionSource=external  InitialCondition=156.9966
  Gain29 : Gain  Gain=0.0000216487318*10^(-9)
  Sum3 : Sum  Inputs=-+-
  k1 : Subsystem
  speed : Subsystem
  to_next_point : Outport
  to_liquid : Outport  Port=2
  wires:
  init_condition_curr_point/1 -> C_steam/2
  speed/1(Out1) -> Sum3/2
  Gain29/1 -> Sum3/3
  Sum3/1 -> C_steam/1
  from_liquid/1 -> Gain29/1
  k1/1(Out1) -> Sum3/1
  C_steam/1 -> k1/2(In2), to_next_point/1, to_liquid/1
  from_T_curr_point/1 -> k1/1(In1)
  EVAP_params/1 -> k1/3(EVAP_params1), speed/3(EVAP_params)
  from_prev_point/1 -> speed/1(In1)
  from_T_prev_point/1 -> speed/2(In2)

== system FRC_0/Bottom RC/Evaporator/T_flue_1 ==
  init_condition_curr_point : Inport
  from_prev_point : Inport  Port=2
  from_side : Inport  Port=3
  Rdg : Gain  Gain=0.47
  Sum2 : Sum  Inputs=++-
  T_flue : Integrator  InitialConditionSource=external  InitialCondition=124.3766
  Vdg/h : Gain  Gain=4.6/1.375
  vdg/h+Rdg : Gain  Gain=4.6/1.375+0.47
  to_next_point : Outport
  to_side : Outport  Port=2
  wires:
  Vdg/h/1 -> Sum2/2
  from_prev_point/1 -> Vdg/h/1
  from_side/1 -> Rdg/1
  vdg/h+Rdg/1 -> Sum2/3
  Sum2/1 -> T_flue/1
  Rdg/1 -> Sum2/1
  init_condition_curr_point/1 -> T_flue/2
  T_flue/1 -> to_next_point/1, vdg/h+Rdg/1, to_side/1

== system FRC_0/Bottom RC/Evaporator/T_flue_2 ==
  init_condition_curr_point : Inport
  from_prev_point : Inport  Port=2
  from_side : Inport  Port=3
  Rdg : Gain  Gain=0.47
  Sum2 : Sum  Inputs=++-
  T_flue : Integrator  InitialConditionSource=external  InitialCondition=124.3766
  Vdg/h : Gain  Gain=4.6/1.375
  vdg/h+Rdg : Gain  Gain=4.6/1.375+0.47
  to_next_point : Outport
  to_side : Outport  Port=2
  wires:
  Vdg/h/1 -> Sum2/2
  from_prev_point/1 -> Vdg/h/1
  from_side/1 -> Rdg/1
  vdg/h+Rdg/1 -> Sum2/3
  Sum2/1 -> T_flue/1
  Rdg/1 -> Sum2/1
  init_condition_curr_point/1 -> T_flue/2
  T_flue/1 -> to_next_point/1, vdg/h+Rdg/1, to_side/1

== system FRC_0/Bottom RC/Evaporator/T_flue_3 ==
  init_condition_curr_point : Inport
  from_prev_point : Inport  Port=2
  from_side : Inport  Port=3
  Rdg : Gain  Gain=0.47
  Sum2 : Sum  Inputs=++-
  T_flue : Integrator  InitialConditionSource=external  InitialCondition=124.3766
  Vdg/h : Gain  Gain=4.6/1.375
  vdg/h+Rdg : Gain  Gain=4.6/1.375+0.47
  to_next_point : Outport
  to_side : Outport  Port=2
  wires:
  Vdg/h/1 -> Sum2/2
  from_prev_point/1 -> Vdg/h/1
  from_side/1 -> Rdg/1
  vdg/h+Rdg/1 -> Sum2/3
  Sum2/1 -> T_flue/1
  Rdg/1 -> Sum2/1
  init_condition_curr_point/1 -> T_flue/2
  T_flue/1 -> to_next_point/1, vdg/h+Rdg/1, to_side/1

== system FRC_0/Bottom RC/Evaporator/T_flue_4 ==
  init_condition_curr_point : Inport
  from_prev_point : Inport  Port=2
  from_side : Inport  Port=3
  Rdg : Gain  Gain=0.47
  Sum2 : Sum  Inputs=++-
  T_flue : Integrator  InitialConditionSource=external  InitialCondition=124.3766
  Vdg/h : Gain  Gain=4.6/1.375
  vdg/h+Rdg : Gain  Gain=4.6/1.375+0.47
  to_next_point : Outport
  to_side : Outport  Port=2
  wires:
  Vdg/h/1 -> Sum2/2
  from_prev_point/1 -> Vdg/h/1
  from_side/1 -> Rdg/1
  vdg/h+Rdg/1 -> Sum2/3
  Sum2/1 -> T_flue/1
  Rdg/1 -> Sum2/1
  init_condition_curr_point/1 -> T_flue/2
  T_flue/1 -> to_next_point/1, vdg/h+Rdg/1, to_side/1

== system FRC_0/Bottom RC/Evaporator/T_liquide_1 ==
  from_side : Inport
  init_condition_curr_point : Inport  Port=2
  from_prev_point : Inport  Port=3
  Ra : Gain  Gain=0.003
  Sum37 : Sum  Inputs=++-
  T_liquide : Integrator  InitialConditionSource=external  InitialCondition=136.285
  va/h+Ra : Gain  Gain=0.003/1.375+0.003
  va/h1 : Gain  Gain=0.003/1.375
  to_side : Outport
  to_next_point : Outport  Port=2
  wires:
  init_condition_curr_point/1 -> T_liquide/2
  va/h1/1 -> Sum37/2
  Sum37/1 -> T_liquide/1
  from_prev_point/1 -> va/h1/1
  Ra/1 -> Sum37/1
  from_side/1 -> Ra/1
  T_liquide/1 -> to_next_point/1, va/h+Ra/1, to_side/1
  va/h+Ra/1 -> Sum37/3

== system FRC_0/Bottom RC/Evaporator/T_liquide_2 ==
  from_side : Inport
  init_condition_curr_point : Inport  Port=2
  from_prev_point : Inport  Port=3
  Ra : Gain  Gain=0.003
  Sum37 : Sum  Inputs=++-
  T_liquide : Integrator  InitialConditionSource=external  InitialCondition=136.285
  va/h+Ra : Gain  Gain=0.003/1.375+0.003
  va/h1 : Gain  Gain=0.003/1.375
  to_side : Outport
  to_next_point : Outport  Port=2
  wires:
  init_condition_curr_point/1 -> T_liquide/2
  va/h1/1 -> Sum37/2
  Sum37/1 -> T_liquide/1
  from_prev_point/1 -> va/h1/1
  Ra/1 -> Sum37/1
  from_side/1 -> Ra/1
  T_liquide/1 -> to_next_point/1, va/h+Ra/1, to_side/1
  va/h+Ra/1 -> Sum37/3

== system FRC_0/Bottom RC/Evaporator/T_liquide_3 ==
  from_side : Inport
  init_condition_curr_point : Inport  Port=2
  from_prev_point : Inport  Port=3
  Ra : Gain  Gain=0.003
  Sum37 : Sum  Inputs=++-
  T_liquide : Integrator  InitialConditionSource=external  InitialCondition=136.285
  va/h+Ra : Gain  Gain=0.003/1.375+0.003
  va/h1 : Gain  Gain=0.003/1.375
  to_side : Outport
  to_next_point : Outport  Port=2
  wires:
  init_condition_curr_point/1 -> T_liquide/2
  va/h1/1 -> Sum37/2
  Sum37/1 -> T_liquide/1
  from_prev_point/1 -> va/h1/1
  Ra/1 -> Sum37/1
  from_side/1 -> Ra/1
  T_liquide/1 -> to_next_point/1, va/h+Ra/1, to_side/1
  va/h+Ra/1 -> Sum37/3

== system FRC_0/Bottom RC/Evaporator/T_liquide_4 ==
  from_side : Inport
  init_condition_curr_point : Inport  Port=2
  from_prev_point : Inport  Port=3
  Ra : Gain  Gain=0.003
  Sum37 : Sum  Inputs=++-
  T_liquide : Integrator  InitialConditionSource=external  InitialCondition=136.285
  va/h+Ra : Gain  Gain=0.003/1.375+0.003
  va/h1 : Gain  Gain=0.003/1.375
  to_side : Outport
  to_next_point : Outport  Port=2
  wires:
  init_condition_curr_point/1 -> T_liquide/2
  va/h1/1 -> Sum37/2
  Sum37/1 -> T_liquide/1
  from_prev_point/1 -> va/h1/1
  Ra/1 -> Sum37/1
  from_side/1 -> Ra/1
  T_liquide/1 -> to_next_point/1, va/h+Ra/1, to_side/1
  va/h+Ra/1 -> Sum37/3

== system FRC_0/Bottom RC/Evaporator/T_side_1 ==
  from_flue : Inport
  init_condition_curr_point : Inport  Port=2
  from_liquide : Inport  Port=3
  Rast : Gain  Gain=0.22
  Rdgst : Gain  Gain=0.008
  Rdgst+Rast : Gain  Gain=0.008+0.22
  Sum2 : Sum  Inputs=++-
  T_side : Integrator  InitialConditionSource=external  InitialCondition=124.3766
  to_flue : Outport
  to_liquide : Outport  Port=2
  wires:
  Rast/1 -> Sum2/2
  from_liquide/1 -> Rast/1
  from_flue/1 -> Rdgst/1
  T_side/1 -> Rdgst+Rast/1, to_liquide/1, to_flue/1
  Rdgst+Rast/1 -> Sum2/3
  Sum2/1 -> T_side/1
  Rdgst/1 -> Sum2/1
  init_condition_curr_point/1 -> T_side/2

== system FRC_0/Bottom RC/Evaporator/T_side_2 ==
  from_flue : Inport
  init_condition_curr_point : Inport  Port=2
  from_liquide : Inport  Port=3
  Rast : Gain  Gain=0.22
  Rdgst : Gain  Gain=0.008
  Rdgst+Rast : Gain  Gain=0.008+0.22
  Sum2 : Sum  Inputs=++-
  T_side : Integrator  InitialConditionSource=external  InitialCondition=124.3766
  to_flue : Outport
  to_liquide : Outport  Port=2
  wires:
  Rast/1 -> Sum2/2
  from_liquide/1 -> Rast/1
  from_flue/1 -> Rdgst/1
  T_side/1 -> Rdgst+Rast/1, to_liquide/1, to_flue/1
  Rdgst+Rast/1 -> Sum2/3
  Sum2/1 -> T_side/1
  Rdgst/1 -> Sum2/1
  init_condition_curr_point/1 -> T_side/2

== system FRC_0/Bottom RC/Evaporator/T_side_3 ==
  from_flue : Inport
  init_condition_curr_point : Inport  Port=2
  from_liquide : Inport  Port=3
  Rast : Gain  Gain=0.22
  Rdgst : Gain  Gain=0.008
  Rdgst+Rast : Gain  Gain=0.008+0.22
  Sum2 : Sum  Inputs=++-
  T_side : Integrator  InitialConditionSource=external  InitialCondition=124.3766
  to_flue : Outport
  to_liquide : Outport  Port=2
  wires:
  Rast/1 -> Sum2/2
  from_liquide/1 -> Rast/1
  from_flue/1 -> Rdgst/1
  T_side/1 -> Rdgst+Rast/1, to_liquide/1, to_flue/1
  Rdgst+Rast/1 -> Sum2/3
  Sum2/1 -> T_side/1
  Rdgst/1 -> Sum2/1
  init_condition_curr_point/1 -> T_side/2

== system FRC_0/Bottom RC/Evaporator/T_side_4 ==
  from_flue : Inport
  init_condition_curr_point : Inport  Port=2
  from_liquide : Inport  Port=3
  Rast : Gain  Gain=0.22
  Rdgst : Gain  Gain=0.008
  Rdgst+Rast : Gain  Gain=0.008+0.22
  Sum2 : Sum  Inputs=++-
  T_side : Integrator  InitialConditionSource=external  InitialCondition=124.3766
  to_flue : Outport
  to_liquide : Outport  Port=2
  wires:
  Rast/1 -> Sum2/2
  from_liquide/1 -> Rast/1
  from_flue/1 -> Rdgst/1
  T_side/1 -> Rdgst+Rast/1, to_liquide/1, to_flue/1
  Rdgst+Rast/1 -> Sum2/3
  Sum2/1 -> T_side/1
  Rdgst/1 -> Sum2/1
  init_condition_curr_point/1 -> T_side/2

== system FRC_0/Bottom RC/Evaporator/T_steam ==
  point_1 : Inport
  point_3 : Inport  Port=2
  point_2 : Inport  Port=3
  point_4 : Inport  Port=4
  Gain : Gain  Gain=1/4
  Sum37 : Sum  Inputs=++++
  to_side : Outport
  wires:
  point_2/1 -> Sum37/2
  point_1/1 -> Sum37/1
  point_3/1 -> Sum37/3
  point_4/1 -> Sum37/4
  Sum37/1 -> Gain/1
  Gain/1 -> to_side/1

== system FRC_0/Bottom RC/RC_buttom/C_liquide_1 ==
  from_steam : Inport
  from_prev_point : Inport  Port=2
  init_condition_curr_point : Inport  Port=3
  Gain18 : Gain  Gain=1.222E-5
  Gain19 : Gain  Gain=0.0002291314/0.5
  Gain22 : Gain  Gain=0.0002291314/0.5-(1.222E-5)*10^(-9)
  Sum2 : Sum  Inputs=-+-
  Tl1 : Integrator  InitialConditionSource=external  InitialCondition=124.3766
  to_steam : Outport
  to_next_point : Outport  Port=2
  wires:
  Gain22/1 -> Sum2/3
  Gain19/1 -> Sum2/2
  Sum2/1 -> Tl1/1
  Tl1/1 -> Gain22/1, to_steam/1, to_next_point/1
  Gain18/1 -> Sum2/1
  init_condition_curr_point/1 -> Tl1/2
  from_prev_point/1 -> Gain19/1
  from_steam/1 -> Gain18/1

== system FRC_0/Bottom RC/RC_buttom/C_liquide_2 ==
  from_steam : Inport
  from_prev_point : Inport  Port=2
  init_condition_curr_point : Inport  Port=3
  Gain18 : Gain  Gain=1.222E-5
  Gain19 : Gain  Gain=0.0002291314/0.5
  Gain22 : Gain  Gain=0.0002291314/0.5-(1.222E-5)*10^(-9)
  Sum2 : Sum  Inputs=-+-
  Tl1 : Integrator  InitialConditionSource=external  InitialCondition=124.3766
  to_steam : Outport
  to_next_point : Outport  Port=2
  wires:
  Gain22/1 -> Sum2/3
  Gain19/1 -> Sum2/2
  Sum2/1 -> Tl1/1
  Tl1/1 -> Gain22/1, to_steam/1, to_next_point/1
  Gain18/1 -> Sum2/1
  init_condition_curr_point/1 -> Tl1/2
  from_prev_point/1 -> Gain19/1
  from_steam/1 -> Gain18/1

== system FRC_0/Bottom RC/RC_buttom/C_liquide_3 ==
  from_steam : Inport
  from_prev_point : Inport  Port=2
  init_condition_curr_point : Inport  Port=3
  Gain18 : Gain  Gain=0.000010734
  Gain19 : Gain  Gain=0.0002291314/0.5
  Gain22 : Gain  Gain=0.0002291314/0.5-(0.000010734)*10^(-9)
  Sum2 : Sum  Inputs=-+-
  Tl1 : Integrator  InitialConditionSource=external  InitialCondition=124.3766
  to_steam : Outport
  to_next_point : Outport  Port=2
  wires:
  Gain22/1 -> Sum2/3
  Gain19/1 -> Sum2/2
  Sum2/1 -> Tl1/1
  Tl1/1 -> Gain22/1, to_steam/1, to_next_point/1
  Gain18/1 -> Sum2/1
  init_condition_curr_point/1 -> Tl1/2
  from_prev_point/1 -> Gain19/1
  from_steam/1 -> Gain18/1

== system FRC_0/Bottom RC/RC_buttom/C_steam_1 ==
  from_T_prev_point : Inport
  from_T_curr_point : Inport  Port=2
  init_condition_curr_point : Inport  Port=3
  from_prev_point : Inport  Port=4
  from_liquid : Inport  Port=5
  Gain29 : Gain  Gain=0.0000216487318*10^(-9)
  Sum3 : Sum  Inputs=-+-
  Tp1 : Integrator  InitialConditionSource=external  InitialCondition=156.9966
  k1 : Subsystem
  speed : Subsystem
  to_next_point : Outport
  to_liquid : Outport  Port=2
  wires:
  init_condition_curr_point/1 -> Tp1/2
  speed/1(Out1) -> Sum3/2
  Gain29/1 -> Sum3/3
  Sum3/1 -> Tp1/1
  from_liquid/1 -> Gain29/1
  k1/1(Out1) -> Sum3/1
  Tp1/1 -> k1/2(In2), to_next_point/1, to_liquid/1
  from_T_curr_point/1 -> k1/1(In1)
  from_T_prev_point/1 -> speed/2(In2)
  from_prev_point/1 -> speed/1(In1)
